simulink model "TempomatMitPI_model"  (R2022b)
settings: Solver=FixedStepAuto  StartTime=0.0  StopTime=tEnd  FixedStep=dtSim  RelTol=1e-8  EnableMultiTasking=on
values from neighbouring files (symbols this model uses):
  A = 2    [TempomatMitPI.m]
  cR = 0.013    [TempomatMitPI.m]
  cW = 0.28    [TempomatMitPI.m]
  g = 9.81    [TempomatMitPI.m]
  KP = 20    [TempomatMitPI.m]
  m = 2000    [TempomatMitPI.m]
  rho = 1.21    [TempomatMitPI.m]
  TI = 60    [TempomatMitPI.m]
settings Model: SimulationMode=accelerator  Creator=Peter  LastModifiedBy=pr1metine
settings SolverCC: AlgebraicLoopSolver=TrustRegion
settings DataIOCC: SaveFormat=Array  SignalLoggingSaveFormat=ModelDataLogs  SaveOutput=off  SignalLogging=off  SaveTime=off  ReturnWorkspaceOutputs=off
settings OptimizationCC: ExpressionDepthLimit=2147483647  LifeSpan=inf
settings DebuggingCC: UnderspecifiedInitializationDetection=Classic  MergeDetectMultiDrivingBlocksExec=none  SolverPrmCheckMsg=warning  FcnCallInpInsideContextMsg=warning  UnconnectedInputMsg=warning  UnconnectedOutputMsg=warning  UnconnectedLineMsg=warning  StateNameClashWarn=warning  SFUnexpectedBacktrackingDiag=warning  SFNoUnconditionalDefaultTransitionDiag=warning  SFExecutionAtInitializationDiag=none  SFMachineParentedDataDiag=warning  ArithmeticOperatorsInVariantConditions=warning
settings HardwareCC: ProdBitPerPointer=32  ProdBitPerSizeT=32  ProdBitPerPtrDiffT=32  ProdLargestAtomicFloat=None  ProdIntDivRoundTo=Undefined  ProdEndianess=Unspecified  ProdWordSize=32  ProdHWDeviceType=32-bit Generic
settings ModelReferenceCC: EnableRefExpFcnMdlSchedulingChecks=on  PropagateSignalLabelsOutOfModel=off
settings SFSimCC: SimUseLocalCustomCode=off  CustomCodeUndefinedFunction=UseInterfaceOnly
settings RTWCC: RTWUseLocalCustomCode=off
settings CodeAppCC: StateflowObjectComments=on
settings GRTTargetCC: TargetLangStandard=C89/C90 (ANSI)  CombineOutputUpdateFcns=off  GRTInterface=on
settings ConfigComp: CovMetricSettings=dw  CovSaveCumulativeToWorkspaceVar=on  CovSaveSingleToWorkspaceVar=on  CovExternalEMLEnable=off

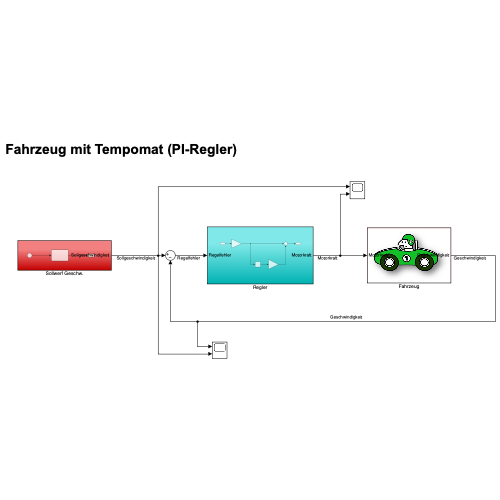
[thumbnail: Simulink's stored preview of the top-level diagram]
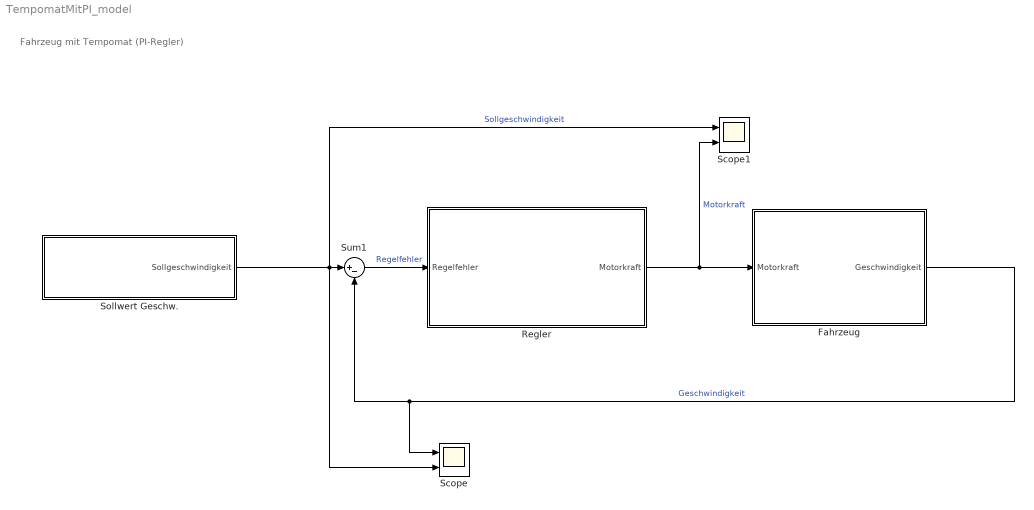
== system TempomatMitPI_model ==
  note: Fahrzeug mit Tempomat (PI-Regler)
  Fahrzeug : Subsystem
      mask Display: image('Auto.jpg'); % Use "Edit Image" on toolstrip to change.
  Regler : Subsystem
  Scope : Scope  NumInputPorts=2
  Scope1 : Scope  NumInputPorts=2
  Sollwert Geschw. : Subsystem
  Sum1 : Sum  Inputs=|+-
  wires:
  Fahrzeug/1(Geschwindigkeit) -> Scope/1, Sum1/2  "Geschwindigkeit"
  Regler/1(Motorkraft) -> Scope1/2, Fahrzeug/1(Motorkraft)  "Motorkraft"
  Sum1/1 -> Regler/1(Regelfehler)  "Regelfehler"
  Sollwert Geschw./1(Sollgeschwindigkeit) -> Scope1/1, Scope/2, Sum1/1  "Sollgeschwindigkeit"

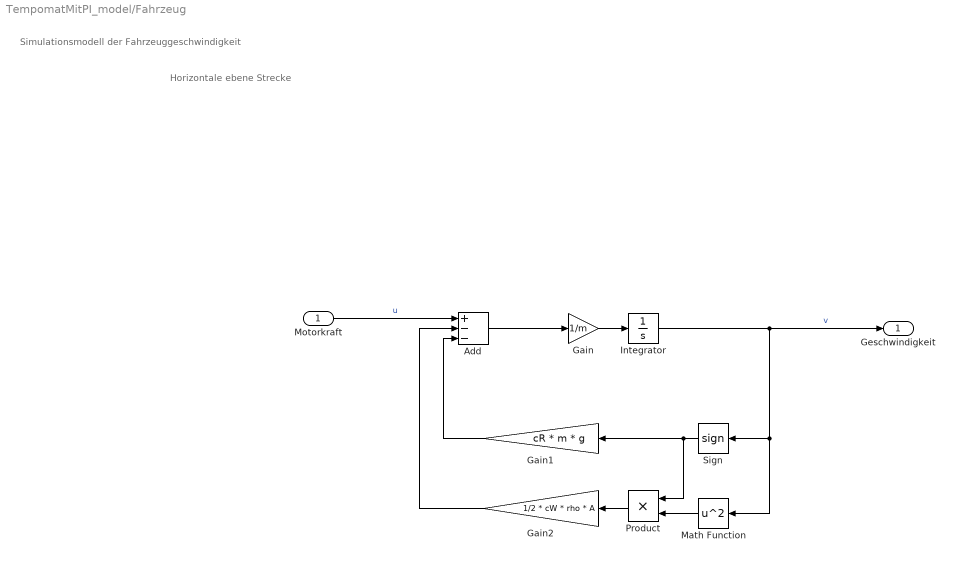
== system TempomatMitPI_model/Fahrzeug ==
  note: Horizontale ebene Strecke
  note: Simulationsmodell der Fahrzeuggeschwindigkeit
  Motorkraft : Inport
  Add : Sum  Inputs=+--
  Gain : Gain  Gain=1/m
  Gain1 : Gain  Gain=cR * m * g
  Gain2 : Gain  Gain=1/2 * cW * rho * A
  Integrator : Integrator
  Math Function : Math  Operator=square
  Product : Product
  Sign : Signum
  Geschwindigkeit : Outport  VectorParamsAs1DForOutWhenUnconnected=off
  wires:
  Integrator/1 -> Math Function/1, Sign/1, Geschwindigkeit/1  "v"
  Gain/1 -> Integrator/1
  Motorkraft/1 -> Add/1  "u"
  Add/1 -> Gain/1
  Sign/1 -> Product/1, Gain1/1
  Gain1/1 -> Add/3
  Math Function/1 -> Product/2
  Product/1 -> Gain2/1
  Gain2/1 -> Add/2

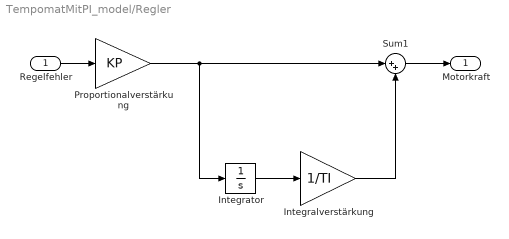
== system TempomatMitPI_model/Regler ==
  Regelfehler : Inport
  Integralverstärkung : Gain  Gain=1/TI
  Integrator : Integrator
  Proportionalverstärkung : Gain  Gain=KP
  Sum1 : Sum  Inputs=|++
  Motorkraft : Outport
  wires:
  Proportionalverstärkung/1 -> Integrator/1, Sum1/1
  Sum1/1 -> Motorkraft/1
  Integrator/1 -> Integralverstärkung/1
  Integralverstärkung/1 -> Sum1/2
  Regelfehler/1 -> Proportionalverstärkung/1

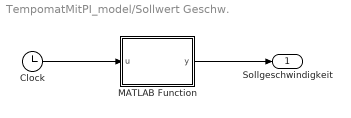
== system TempomatMitPI_model/Sollwert Geschw. ==
  Clock : Clock
  MATLAB Function : MATLAB Function  TreatAsAtomicUnit=on
  Sollgeschwindigkeit : Outport
  wires:
  MATLAB Function/1(y) -> Sollgeschwindigkeit/1
  Clock/1 -> MATLAB Function/1(u)

== matlab function TempomatMitPI_model/Sollwert Geschw./MATLAB Function ==
  data: u input; y output
function y = fcn(u)
    if u < 100
        y = 0;
    elseif u < 1000
        y = 40;
    elseif u < 2000
        y = 20;
    elseif u < 2500
        y = 10;
    else
        y = 40;
    end
end
